simulink model "Sistema_Seguimiento_Tipo1_Con_Planta_Tipo_0"  (R2023a)
settings: Solver=VariableStepAuto  StartTime=0.0  StopTime=Tiempo_Sim  RelTol=1e-3  EnableMultiTasking=on
values from neighbouring files (symbols this model uses):
  A = flip(fliplr(A))    [Ejercicio_Ackerman.m]
  B = flip(B)    [Ejercicio_Ackerman.m]
  C = fliplr(C)    [Ejercicio_Ackerman.m]
  Init_cond = 0    [Ejercicio_Ackerman.m]
  K = acker(A,B,PLC)    [Ejercicio_Ackerman.m]
  kr = 1 / (C * inv(-A + B*K) * B)    [Ejercicio_Ackerman.m]
undefined symbols (not defined in the file or in its folder): D
libraries: simulink x1
settings Model: Creator=adrie  LastModifiedBy=adrie
settings SolverCC: AlgebraicLoopSolver=TrustRegion
settings DataIOCC: ReturnWorkspaceOutputs=off
settings OptimizationCC: LifeSpan=inf
settings DebuggingCC: UnconnectedInputMsg=warning  UnconnectedOutputMsg=warning  UnconnectedLineMsg=warning  SFUnexpectedBacktrackingDiag=warning  SFNoUnconditionalDefaultTransitionDiag=warning  ArithmeticOperatorsInVariantConditions=warning
settings ModelReferenceCC: EnableRefExpFcnMdlSchedulingChecks=on
settings SFSimCC: SimUseLocalCustomCode=off  CustomCodeUndefinedFunction=UseInterfaceOnly
settings RTWCC: RTWUseLocalCustomCode=off
settings CodeAppCC: StateflowObjectComments=on
settings GRTTargetCC: TargetLangStandard=C89/C90 (ANSI)
settings ConfigComp: CovMetricSettings=dw  CovSaveCumulativeToWorkspaceVar=on  CovSaveSingleToWorkspaceVar=on  CovExternalEMLEnable=off

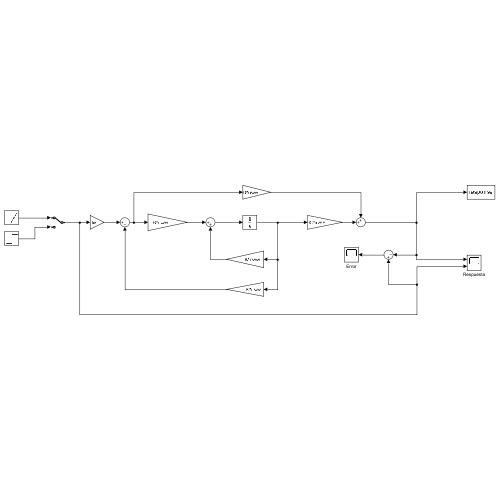
[thumbnail: Simulink's stored preview of the top-level diagram]
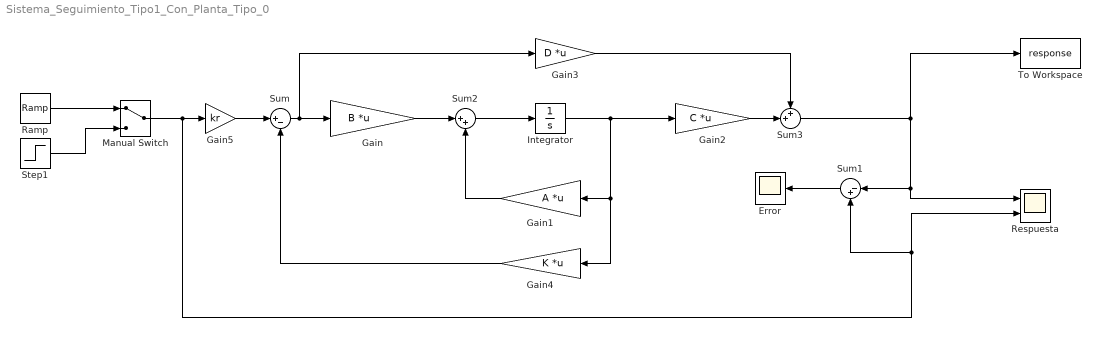
== system Sistema_Seguimiento_Tipo1_Con_Planta_Tipo_0 ==
  Error : Scope
  Gain : Gain  Gain=B  Multiplication=Matrix(K*u) (u vector)
  Gain1 : Gain  Gain=A  Multiplication=Matrix(K*u) (u vector)
  Gain2 : Gain  Gain=C  Multiplication=Matrix(K*u) (u vector)
  Gain3 : Gain  Gain=D  Multiplication=Matrix(K*u) (u vector)
  Gain4 : Gain  Gain=K  Multiplication=Matrix(K*u) (u vector)
  Gain5 : Gain  Gain=kr
  Integrator : Integrator  InitialCondition=Init_cond
  Manual Switch : ManualSwitch
  Ramp : simulink/Sources/Ramp  slope=1  start=0  InitialOutput=0
  Respuesta : Scope  NumInputPorts=2
  Step1 : Step  Time=0  SampleTime=0
  Sum : Sum  Inputs=|+-
  Sum1 : Sum  Inputs=|-+
  Sum2 : Sum  Inputs=|++
  Sum3 : Sum  Inputs=++|
  To Workspace : ToWorkspace  VariableName=response  SaveFormat=Timeseries  SampleTime=-1
      settings: Save2DSignal=2-D array (concatenate along first dimension)
  wires:
  Gain/1 -> Sum2/1
  Sum2/1 -> Integrator/1
  Gain1/1 -> Sum2/2
  Integrator/1 -> Gain2/1, Gain4/1, Gain1/1
  Gain2/1 -> Sum3/2
  Gain3/1 -> Sum3/1
  Sum/1 -> Gain3/1, Gain/1
  Gain4/1 -> Sum/2
  Gain5/1 -> Sum/1
  Sum3/1 -> To Workspace/1, Sum1/1, Respuesta/1
  Ramp/1 -> Manual Switch/1
  Step1/1 -> Manual Switch/2
  Manual Switch/1 -> Sum1/2, Respuesta/2, Gain5/1
  Sum1/1 -> Error/1
